simulink model "full_maneuver_single_veh"  (R2020a)
settings: Solver=VariableStepAuto  StartTime=0.0  StopTime=90  FixedStep=0.1  MaxStep=5e-2  RelTol=1e-3
InitFcn:
  | totalVehicles = 5;
  | if exist('vehStatesBus', 'var')==0
  | load vehBuses
  | end
  | if exist('vehErrorsBus', 'var')==0
  | load vehBuses
  | end
libraries: simulink x69, powerlib_meascontrol x6, autolibshared x6, dspsigops x3, eeGeneralControl x2
(part 2 of 6)

== system full_maneuver_single_veh/Lo ==
  allVehicles : Inport
  Constant{,1,3,6} (4 alike) : Constant  Value=0
  Gain : Gain  Gain=m/2
  Regular Vehicle Following : Subsystem
  Terminator{,1..3,9..12} (8 alike) : Terminator
  Transfer Fcn : TransferFcn  Denominator=[tau 1]
  Transport Delay1 : TransportDelay  DelayTime=0.01
  Vehicle Body 3DOF Single Track : autolibshared/Vehicle Body 3DOF Single Track  trackMode=Single (bicycle)  inputMode=External longitudinal forces  frontSteerMode=on  rearSteerMode=off  windMode=off  muMode=off  extFMode=off  extMMode=off  extXo=off  extpsio=off  extxdoto=off  extro=off  extYo=off  extTamb=off  extydoto=off  aMode=2  NF=2  NR=2  m=m  a=lf  b=lr  h=0.35  X_o=x0  xdot_o=vx0  CalphaMode=off  sigmaMode=on  d=0  w=[1.4,1.4]  Cy_f=12e3  Cy_r=11e3  sigma_f=.1  sigma_r=.1  alpha_f_brk=[-.1 .1]  Cy_f_data=[-9e3 9e3]  alpha_r_brk=[-.1 .1]  Cy_r_data=[-9e3 9e3]  Y_o=y0  ydot_o=0  Izz=4000  psi_o=0  r_o=0  Af=2  Cd=.3  Cl=.1  Cpm=.1  beta_w=[0:0.01:0.3]  Cs=[0:0.03:0.9]  Cym=[0:0.01:0.3]  Pabs=101325  Tair=273  g=9.81  mu=1  xdot_tol=.01  Fznom=5000  Fxtire_sat=7e4  Fytire_sat=7e4  longOff=0  latOff=0  vertOff=0  wrapAng=off
      settings: SourceProductBaseCode=PW,MT,VE,VP
  findLeader : Subsystem
  states routing : Subsystem
  states : Outport  VectorParamsAs1DForOutWhenUnconnected=off
  errors : Outport  Port=2  VectorParamsAs1DForOutWhenUnconnected=off
  gap : Outport  Port=3  VectorParamsAs1DForOutWhenUnconnected=off
  wires:
  Transfer Fcn/1 -> Gain/1
  findLeader/1(leader) -> Regular Vehicle Following/2(leader)
  Regular Vehicle Following/4(leaderInRange) -> Terminator3/1
  Constant3/1 -> Regular Vehicle Following/4(extraSpaceFlag)
  Constant/1 -> states routing/1(delta), Vehicle Body 3DOF Single Track/1  "delta"
  Regular Vehicle Following/2(errors) -> errors/1
  Regular Vehicle Following/1(u) -> Transport Delay1/1  "u"
  findLeader/2(leaderChange) -> Regular Vehicle Following/3(leaderChange)
  Transport Delay1/1 -> states routing/3(u), Transfer Fcn/1
  states routing/2(observedStates) -> Regular Vehicle Following/1(ego), findLeader/1(ego), states/1
  Vehicle Body 3DOF Single Track/1 -> states routing/2(Info)
  Gain/1 -> Vehicle Body 3DOF Single Track/3, Vehicle Body 3DOF Single Track/2
  allVehicles/1 -> findLeader/2(all)
  Regular Vehicle Following/3(gap) -> gap/1
  Constant1/1 -> findLeader/4(state)
  Constant6/1 -> findLeader/3(lcFlag)
  states routing/1(latStates) -> Terminator1/1
  Vehicle Body 3DOF Single Track/2 -> Terminator2/1
  Vehicle Body 3DOF Single Track/5 -> Terminator10/1
  Vehicle Body 3DOF Single Track/3 -> Terminator/1
  Vehicle Body 3DOF Single Track/6 -> Terminator11/1
  Vehicle Body 3DOF Single Track/7 -> Terminator12/1
  Vehicle Body 3DOF Single Track/4 -> Terminator9/1

== system full_maneuver_single_veh/Subsystem ==
  note: Lane change not yet completed
  laneChangeIntention : Inport
  platoonState : Inport  Port=2
  AND : Logic  IconShape=distinctive  AllPortsSameDT=off  OutDataTypeStr=boolean
  Compare To Constant : simulink/Logic and Bit Operations/Compare To Constant  relop=<  const=5  OutDataTypeStr=boolean
  Selector : Selector  InputPortWidth=1  IndexOptions=Index vector (dialog)  Indices=[1]  OutputSizes=1
  gapRequest : Outport
  wires:
  laneChangeIntention/1 -> AND/1
  platoonState/1 -> Selector/1
  Selector/1 -> Compare To Constant/1
  AND/1 -> gapRequest/1
  Compare To Constant/1 -> AND/2

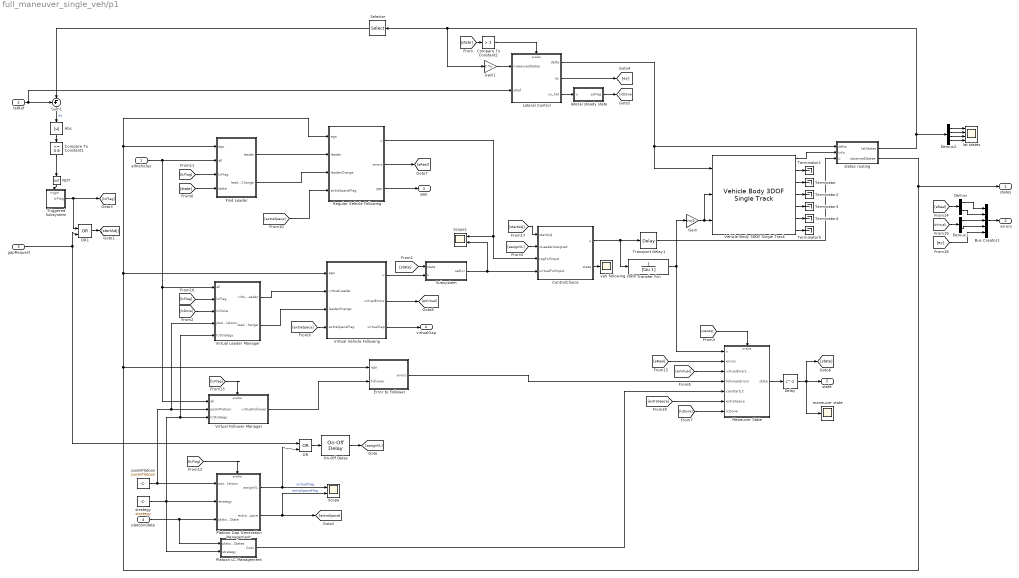
== system full_maneuver_single_veh/p1 ==
  allVehicles : Inport
  latRef : Inport  Port=2
  gapRequest : Inport  Port=3
  platoonState : Inport  Port=4
  Abs : Abs
  Bus Creator1 : BusCreator  Inputs=5  OutDataTypeStr=Bus: vehErrorsBus  NonVirtualBus=on
      settings: InheritFromInputs=off
  Compare To Constant1 : simulink/Logic and Bit Operations/Compare To Constant  relop=<=  const=0.8  OutDataTypeStr=boolean
  Compare To Constant2 : simulink/Logic and Bit Operations/Compare To Constant  relop=>  const=3  OutDataTypeStr=boolean
  ControlChoice : Stateflow chart  TreatAsAtomicUnit=on
  Delay : Delay
  Demux : Demux  Outputs=2
  Demux1 : Demux  Outputs=2
  Demux2 : Demux
  Error to Follower : Subsystem
  Find Leader : Subsystem
  Gain : Gain  Gain=m/2
  Gain1 : Gain  Gain=C  Multiplication=Matrix(K*u)
  Lateral Control : Subsystem
  Maneuver State : Subsystem
  NOT : Logic  Operator=NOT  IconShape=distinctive  AllPortsSameDT=off  OutDataTypeStr=boolean
  OR : Logic  Operator=OR  IconShape=distinctive  AllPortsSameDT=off  OutDataTypeStr=boolean
  OR1 : Logic  Operator=OR  IconShape=distinctive  AllPortsSameDT=off  OutDataTypeStr=boolean
  On-Off Delay : eeGeneralControl/On-Off Delay  LabelModeActiveChoice=Continuous  Td_on=0.1  Td_off=1  IC=0  Ts=0
      settings: SourceProductBaseCode=PS
  Platoon Gap Generation Management : Subsystem
  Platoon LC Management : Subsystem
  Regular Vehicle Following : Subsystem
  Scope : Scope  NumInputPorts=2
  Scope1 : Scope  NumInputPorts=2
  Selector : Selector  InputPortWidth=4  IndexOptions=Index vector (dialog)  Indices=1  OutputSizes=1
  Subsystem : Subsystem
  Sum1 : Sum  Inputs=+-|
  Terminator{,1..5} (6 alike) : Terminator
  Transfer Fcn : TransferFcn  Denominator=[tau 1]
  Transport Delay1 : TransportDelay  DelayTime=0.01
  Triggered Subsystem : Subsystem  TreatAsAtomicUnit=on
  Vehicle Body 3DOF Single Track : autolibshared/Vehicle Body 3DOF Single Track  trackMode=Single (bicycle)  inputMode=External longitudinal forces  frontSteerMode=on  rearSteerMode=off  windMode=off  muMode=off  extFMode=off  extMMode=off  extXo=off  extpsio=off  extxdoto=off  extro=off  extYo=off  extTamb=off  extydoto=off  aMode=2  NF=2  NR=2  m=m  a=lf  b=lr  h=0.35  X_o=x0  xdot_o=vx0  CalphaMode=off  sigmaMode=on  d=0  w=[1.4,1.4]  Cy_f=12e3  Cy_r=11e3  sigma_f=.1  sigma_r=.1  alpha_f_brk=[-.1 .1]  Cy_f_data=[-9e3 9e3]  alpha_r_brk=[-.1 .1]  Cy_r_data=[-9e3 9e3]  Y_o=y0  ydot_o=0  Izz=4000  psi_o=0  r_o=0  Af=2  Cd=.3  Cl=.1  Cpm=.1  beta_w=[0:0.01:0.3]  Cs=[0:0.03:0.9]  Cym=[0:0.01:0.3]  Pabs=101325  Tair=273  g=9.81  mu=1  xdot_tol=.01  Fznom=5000  Fxtire_sat=7e4  Fytire_sat=7e4  longOff=0  latOff=0  vertOff=0  wrapAng=off
      settings: SourceProductBaseCode=PW,MT,VE,VP
  Virtual Follower Manager : Subsystem  TreatAsAtomicUnit=on
  Virtual Leader Manager : Subsystem  TreatAsAtomicUnit=on
  Virtual Vehicle Following : Subsystem  TreatAsAtomicUnit=on
  lat states : Scope  NumInputPorts=4
  lateral steady state : Subsystem
  maneuver state : Scope
  posInPlatoon : Constant  Value=posInPlatoon
  states routing : Subsystem
  strategy : Constant  Value=strategy
  veh following state : Scope
  states : Outport  VectorParamsAs1DForOutWhenUnconnected=off
  errors : Outport  Port=2  VectorParamsAs1DForOutWhenUnconnected=off
  gap : Outport  Port=3  VectorParamsAs1DForOutWhenUnconnected=off
  virtualGap : Outport  Port=4  VectorParamsAs1DForOutWhenUnconnected=off
  state : Outport  Port=5  VectorParamsAs1DForOutWhenUnconnected=off
  wires:
  [extraSpace] -> Maneuver State/6(extraSpace)
  [eReal] -> Maneuver State/2(errors)
  [eVirtual] -> Maneuver State/3(virtualErrors)
  [lcDone] -> Maneuver State/7(lcDone)
  [startAdj] -> Maneuver State/Enable
  Platoon LC Management/1(Out1) -> Maneuver State/5(canStartLC)
  Error to Follower/1(errors) -> Maneuver State/4(followerErrors)
  Maneuver State/1(state) -> Delay/1
  [lcFlag] -> Virtual Leader Manager/2(lcFlag)
  [lcDone] -> Virtual Leader Manager/3(lcDone)
  [lcFlag] -> Virtual Follower Manager/Enable
  [lcFlag] -> Platoon Gap Generation Management/Enable
  [lcFlag] -> Find Leader/3(lcFlag)
  [extraSpace] -> Regular Vehicle Following/4(extraSpaceFlag)
  [extraSpace] -> Virtual Vehicle Following/4(extraSpaceFlag)
  Platoon Gap Generation Management/1(assignVL) -> OR/2, Scope/1  "virtualFlag"
  [assignVL] -> ControlChoice/2(vLeaderAssigned)
  gapRequest/1 -> OR/1, OR1/2
  Triggered Subsystem/1(lcFlag) -> [lcFlag], OR1/1
  Regular Vehicle Following/2(errors) -> [eReal]
  Virtual Vehicle Following/2(virtualErrors) -> [eVirtual]
  Virtual Leader Manager/2(leaderChange) -> Virtual Vehicle Following/3(leaderChange)
  Compare To Constant1/1 -> NOT/1
  [startAdj] -> ControlChoice/1(startAdj)
  Virtual Leader Manager/1(virtualLeader) -> Virtual Vehicle Following/2(virtualLeader)
  posInPlatoon/1 -> Virtual Leader Manager/4(posInPlatoon), Virtual Follower Manager/2(posInPlatoon), Platoon Gap Generation Management/1(posInPlatoon)
  [state] -> Subsystem/1(state)
  Find Leader/1(leader) -> Regular Vehicle Following/2(leader)
  Subsystem/1(sat(u)) -> ControlChoice/4(virtualFollInput), Scope1/2
  Find Leader/2(leaderChange) -> Regular Vehicle Following/3(leaderChange)
  Sum1/1 -> Abs/1  "ey"
  Transfer Fcn/1 -> Gain/1, Maneuver State/1(u)
  states routing/2(observedStates) -> states/1, Virtual Vehicle Following/1(ego), Regular Vehicle Following/1(ego), Find Leader/1(ego), Error to Follower/1(ego)
  latRef/1 -> Lateral Control/2(yRef), Sum1/1
  Vehicle Body 3DOF Single Track/3 -> Terminator/1
  Vehicle Body 3DOF Single Track/1 -> states routing/2(Info)
  Gain/1 -> Vehicle Body 3DOF Single Track/3, Vehicle Body 3DOF Single Track/2
  Platoon Gap Generation Management/2(extraSpace) -> Scope/2, [extraSpace]  "extraSpaceFlag"
  Abs/1 -> Compare To Constant1/1
  allVehicles/1 -> Find Leader/2(all), Virtual Leader Manager/1(all), Virtual Follower Manager/1(all)
  Regular Vehicle Following/3(gap) -> gap/1
  Regular Vehicle Following/1(u) -> ControlChoice/3(regFollInput), Scope1/1
  Virtual Vehicle Following/1(u) -> Subsystem/2(u)
  Compare To Constant2/1 -> Lateral Control/Enable
  Virtual Vehicle Following/3(virtualGap) -> virtualGap/1
  [state] -> Compare To Constant2/1
  platoonState/1 -> Platoon Gap Generation Management/3(platoonState), Platoon LC Management/1(platoonStates)
  Delay/1 -> state/1, [state], maneuver state/1
  strategy/1 -> Virtual Leader Manager/5(lcStrategy), Virtual Follower Manager/3(lcStrategy), Platoon LC Management/2(strategy), Platoon Gap Generation Management/2(strategy)
  [state] -> Find Leader/4(state)
  OR1/1 -> [startAdj]
  states routing/1(latStates) -> Demux2/1, Selector/1, Gain1/1
  Gain1/1 -> Lateral Control/1(measuredStates)
  NOT/1 -> Triggered Subsystem/Trigger
  Lateral Control/3(vy_hat) -> lateral steady state/1(u)
  lateral steady state/1(ssFlag) -> [lcDone]
  Lateral Control/2(ey) -> [ey]
  [eVirtual] -> Demux1/1
  [eReal] -> Demux/1
  Demux/1 -> Bus Creator1/1
  Demux/2 -> Bus Creator1/2
  Demux1/1 -> Bus Creator1/3
  Demux1/2 -> Bus Creator1/4
  [ey] -> Bus Creator1/5
  Bus Creator1/1 -> errors/1
  OR/1 -> On-Off Delay/1
  Lateral Control/1(delta) -> Vehicle Body 3DOF Single Track/1, states routing/1(delta)
  Demux2/1 -> lat states/1
  Demux2/2 -> lat states/2
  Demux2/3 -> lat states/3
  Demux2/4 -> lat states/4
  Selector/1 -> Sum1/2
  Vehicle Body 3DOF Single Track/2 -> Terminator1/1
  Vehicle Body 3DOF Single Track/4 -> Terminator2/1
  Vehicle Body 3DOF Single Track/5 -> Terminator3/1
  Vehicle Body 3DOF Single Track/6 -> Terminator4/1
  Vehicle Body 3DOF Single Track/7 -> Terminator5/1
  ControlChoice/1(u) -> Transfer Fcn/1, Transport Delay1/1
  Virtual Follower Manager/1(virtualFollower) -> Error to Follower/2(follower)
  ControlChoice/2(state) -> veh following state/1
  Transport Delay1/1 -> states routing/3(u)
  On-Off Delay/1 -> [assignVL]

== system full_maneuver_single_veh/Fd/Error to Follower ==
  ego : Inport
  follower : Inport  Port=2
  Bus Selector : BusSelector  OutputSignals=X,Xdot
  Bus Selector1 : BusSelector  OutputSignals=X,Xdot
  Multiply : Product
  Mux : Mux  Inputs=2
  Sum : Sum  Inputs=-+|
  Sum1 : Sum  Inputs=++|
  Sum2 : Sum  Inputs=+-|
  Sum3 : Sum  Inputs=|++
  Sum4 : Sum  Inputs=-+|
  d0 : Constant  Value=d0
  h : Constant  Value=h
  vLen : Constant  Value=lr+lf
  errors : Outport  VectorParamsAs1DForOutWhenUnconnected=off
  wires:
  d0/1 -> Sum3/2  "gap at  standstill"
  h/1 -> Multiply/2  "time headway"
  Sum2/1 -> Mux/1
  Bus Selector1/1 -> Sum/2  "<X>"
  Sum1/1 -> Sum/1  "x (front bumber)"
  Sum3/1 -> Sum2/2  "desired  gap"
  Bus Selector/1 -> Sum1/2  "<X>"
  Sum/1 -> Sum2/1  "gap"
  Multiply/1 -> Sum3/1
  vLen/1 -> Sum1/1
  follower/1 -> Bus Selector/1
  ego/1 -> Bus Selector1/1
  Bus Selector/2 -> Sum4/1, Multiply/1  "<Xdot>"
  Bus Selector1/2 -> Sum4/2  "<Xdot>"
  Sum4/1 -> Mux/2
  Mux/1 -> errors/1

== system full_maneuver_single_veh/Fd/Find Leader ==
  ego : Inport
  all : Inport  Port=2
  lcFlag : Inport  Port=3
  state : Inport  Port=4
  Compare To Constant : simulink/Logic and Bit Operations/Compare To Constant  relop=~=  const=4  OutDataTypeStr=boolean
  Detect Change : simulink/Logic and Bit Operations/Detect Change  vinit=0  OutDataTypeStr=boolean
  NOT : Logic  Operator=NOT  IconShape=distinctive  AllPortsSameDT=off  OutDataTypeStr=boolean
  OR : Logic  Operator=OR  IconShape=distinctive  AllPortsSameDT=off  OutDataTypeStr=boolean
  Selector : Selector  InputPortWidth=totalVehicles+1  IndexOptions=Index vector (port)  Indices=[1]  OutputSizes=1
  Subsystem : Subsystem
  Vector Concatenate : Concatenate
  farAwayVeh : Subsystem
  realLeaderIdx : Scope
  leader : Outport  VectorParamsAs1DForOutWhenUnconnected=off
  leaderChange : Outport  Port=2  InitialOutput=1  VectorParamsAs1DForOutWhenUnconnected=off
  wires:
  Compare To Constant/1 -> OR/2
  state/1 -> Compare To Constant/1
  ego/1 -> Subsystem/1(ego), farAwayVeh/1(ego)
  all/1 -> Vector Concatenate/1, Subsystem/2(all)
  Subsystem/1(idx) -> realLeaderIdx/1, Selector/2, Detect Change/1
  OR/1 -> Subsystem/Enable
  lcFlag/1 -> NOT/1
  NOT/1 -> OR/1
  Selector/1 -> leader/1
  farAwayVeh/1(Out1) -> Vector Concatenate/2
  Vector Concatenate/1 -> Selector/1
  Detect Change/1 -> leaderChange/1

== system full_maneuver_single_veh/Fd/Lateral Control ==
  measuredStates : Inport
  yRef : Inport  Port=2
  Enable : EnablePort
  Demux2 : Demux
  Full State Observer : Subsystem  Commented=on
  Gain : Gain  Gain=5
  Gain1 : Gain  Gain=Klat  Multiplication=Matrix(K*u)
  Integrator : Integrator  InitialCondition=y0
  Pad : dspsigops/Pad  padAlong=Columns  dimsToPad=1  valSrc=Specify via dialog  padVal=0  spec=Output size  padNumOutRowsSpecMethod=User-specified  numOutRows=4  padNumOutColsSpecMethod=User-specified  numOutCols=1  isVarDimsMode=off  padBeginning=0  padEnd=0  outSizeMode=User-specified  outSize=1  padSigAt=End  trunc_flag=None  roundingMode=Floor  overflowMode=off  truncOrWrapMode=Truncate  wrap_flag=None
      settings: SourceProductBaseCode=DS
  Rate Limiter : RateLimiter  RisingSlewLimit=maxDeltaDot  FallingSlewLimit=-maxDeltaDot  SampleTimeMode=inherited
  Saturation : Saturate  UpperLimit=maxDelta  LowerLimit=-maxDelta
  Saturation1 : Saturate  UpperLimit=2  LowerLimit=-2
  Scope : Scope  NumInputPorts=4
  Scope1 : Scope  NumInputPorts=2
  Selector : Selector  InputPortWidth=4  IndexOptions=Index vector (dialog)  Indices=[1]  OutputSizes=1
  Sum : Sum  Inputs=|+-
  Sum2 : Sum  Inputs=|+-
  delta : Outport  VectorParamsAs1DForOutWhenUnconnected=off
  ey : Outport  Port=2  VectorParamsAs1DForOutWhenUnconnected=off
  vy_hat : Outport  Port=3  InitialOutput=0.3  VectorParamsAs1DForOutWhenUnconnected=off
  wires:
  Selector/1 -> ey/1
  Saturation1/1 -> Integrator/1
  Gain/1 -> Saturation1/1
  measuredStates/1 -> Sum/2, Demux2/1, Full State Observer/1(measuredOutputs)  "estStates"
  yRef/1 -> Sum2/1
  Demux2/3 -> Scope/3
  Saturation/1 -> Rate Limiter/1
  Sum2/1 -> Gain/1
  Demux2/2 -> Scope/2, vy_hat/1
  Demux2/4 -> Scope/4
  Pad/1 -> Sum/1
  Sum/1 -> Gain1/1, Selector/1
  Gain1/1 -> Saturation/1, Scope1/2
  Integrator/1 -> Pad/1, Sum2/2
  Demux2/1 -> Scope/1
  Rate Limiter/1 -> delta/1, Scope1/1, Full State Observer/2(delta)  "delta"

== system full_maneuver_single_veh/Fd/Maneuver State ==
  note: States are:
      | 0 - Lane keeping
      | 1 - Longitudinal Adjustment
      | 2 - Steady State
      | 3 - Safe to LC
      | 4 - Performing LC
      | 5 - LC is done
      | 6 - Long Adj done
  u : Inport
  errors : Inport  Port=2
  virtualErrors : Inport  Port=3
  followerErrors : Inport  Port=4
  canStartLC : Inport  Port=5
  extraSpace : Inport  Port=6
  lcDone : Inport  Port=7
  Enable : EnablePort
  AND : Logic  IconShape=distinctive  AllPortsSameDT=off  OutDataTypeStr=boolean
  AND1 : Logic  IconShape=distinctive  AllPortsSameDT=off  OutDataTypeStr=boolean
  AND2 : Logic  Inputs=3  IconShape=distinctive  AllPortsSameDT=off  OutDataTypeStr=boolean
  AND{3..7} (5 alike) : Logic  IconShape=distinctive  AllPortsSameDT=off  OutDataTypeStr=fixdt(1,16)
  Constant : Constant
  Data Type Conversion : DataTypeConversion  OutMin=0  OutMax=1  OutDataTypeStr=fixdt(1,16)
  Memory : Memory
  NOT1 : Logic  Operator=NOT  IconShape=distinctive  AllPortsSameDT=off  OutDataTypeStr=boolean
  On Delay : powerlib_meascontrol/Logic/On Delay  DelayType=On delay  delay=1  ic=0  Ts=0
  On Delay1 : powerlib_meascontrol/Logic/On Delay  DelayType=On delay  delay=0.2  ic=0  Ts=0
  Scope : Scope  NumInputPorts=5
  Sum : Sum  Inputs=++++++
  Triggered Subsystem : Subsystem  TreatAsAtomicUnit=on
  Triggered Subsystem1 : Subsystem  TreatAsAtomicUnit=on
  safeErrors : Subsystem
  safeErrors1 : Subsystem
  safeErrors2 : Subsystem
  steadyState : Subsystem
  state : Outport  InitialOutput=0  VectorParamsAs1DForOutWhenUnconnected=off
  wires:
  u/1 -> steadyState/1(u)
  AND1/1 -> AND/1, AND2/1  "steady state"
  steadyState/1(ssFlag) -> AND1/1
  safeErrors2/1(safetyFlag) -> AND2/2
  Triggered Subsystem1/1(Out1) -> Memory/1
  NOT1/1 -> On Delay1/1
  On Delay/1 -> AND2/3
  extraSpace/1 -> On Delay/1, NOT1/1
  safeErrors1/1(safetyFlag) -> AND1/2
  AND2/1 -> Triggered Subsystem1/Trigger
  On Delay1/1 -> AND/2
  followerErrors/1 -> safeErrors/1(errors)
  errors/1 -> safeErrors1/1(errors)
  virtualErrors/1 -> safeErrors2/1(errors)
  Triggered Subsystem/1(Out1) -> Sum/6
  canStartLC/1 -> AND5/2
  lcDone/1 -> AND6/2
  AND7/1 -> Scope/5, Triggered Subsystem/Trigger
  Data Type Conversion/1 -> Sum/1
  AND/1 -> AND7/2
  AND6/1 -> AND7/1, Sum/5, Scope/4
  Constant/1 -> AND3/1, Data Type Conversion/1
  AND5/1 -> Sum/4, Scope/3, AND6/1
  AND3/1 -> Sum/2, Scope/1, AND4/1
  Sum/1 -> state/1
  safeErrors/1(safetyFlag) -> AND4/2
  AND4/1 -> Sum/3, Scope/2, AND5/1
  Memory/1 -> AND3/2

== system full_maneuver_single_veh/Fd/Platoon Gap Generation Management ==
  posInPlatoon : Inport
  strategy : Inport  Port=2
  platoonState : Inport  Port=3
  Enable : EnablePort
  Scope : Scope  NumInputPorts=2
  assignExtraSpace : MATLAB Function  TreatAsAtomicUnit=on
  assignvirtualLeader : MATLAB Function  TreatAsAtomicUnit=on
  assignVL : Outport  VectorParamsAs1DForOutWhenUnconnected=off
  extraSpace : Outport  Port=2  VectorParamsAs1DForOutWhenUnconnected=off
  wires:
  assignvirtualLeader/1(virtualLeaderFlag) -> assignVL/1, Scope/1
  platoonState/1 -> assignExtraSpace/3(platoonState), assignvirtualLeader/3(platoonState)
  posInPlatoon/1 -> assignExtraSpace/2(posInPlatoon), assignvirtualLeader/2(posInPlatoon)
  strategy/1 -> assignExtraSpace/1(strategy), assignvirtualLeader/1(strategy)
  assignExtraSpace/1(extraSpaceFlag) -> extraSpace/1, Scope/2

== system full_maneuver_single_veh/Fd/Platoon LC Management ==
  platoonStates : Inport
  strategy : Inport  Port=2
  Compare To Constant : simulink/Logic and Bit Operations/Compare To Constant  relop=>  const=1  OutDataTypeStr=boolean
  Compare To Constant1 : simulink/Logic and Bit Operations/Compare To Constant  relop=>  const=2  OutDataTypeStr=boolean
  OR : Logic  Operator=OR  IconShape=distinctive  AllPortsSameDT=off  OutDataTypeStr=boolean
  Selector : Selector  IndexOptions=Index vector (port)  Indices=[1 3]  OutputSizes=1
  Width : Width
  Out1 : Outport  VectorParamsAs1DForOutWhenUnconnected=off
  wires:
  Compare To Constant1/1 -> OR/1
  Selector/1 -> Compare To Constant1/1
  Width/1 -> Selector/2
  platoonStates/1 -> Selector/1, Width/1
  OR/1 -> Out1/1
  Compare To Constant/1 -> OR/2
  strategy/1 -> Compare To Constant/1

== system full_maneuver_single_veh/Fd/Regular Vehicle Following ==
  ego : Inport
  leader : Inport  Port=2
  leaderChange : Inport  Port=3
  extraSpaceFlag : Inport  Port=4
  Bus Selector : BusSelector  OutputSignals=u
  Compute Errors : Subsystem
  Constant : Constant  Value=0
  Define Desired Distance : Subsystem
  Rate Limiter : RateLimiter  RisingSlewLimit=maxJerk  FallingSlewLimit=minJerk  SampleTimeMode=inherited
  Rate Limiter1 : RateLimiter  RisingSlewLimit=maxComfJerk  FallingSlewLimit=minComfJerk  SampleTimeMode=inherited
  Switch : Switch  Criteria=u2 > Threshold
  Switch1 : Switch  Criteria=u2 > Threshold
  Veh Following : Subsystem  TreatAsAtomicUnit=on
  Velocity Control : Subsystem  TreatAsAtomicUnit=on
  Velocity Error : Subsystem
  comf saturation : Saturate  UpperLimit=maxComfAccel  LowerLimit=minComfAccel
  errorScope : Scope
  freeFlowVel : Constant  Value=freeFlowVel
  safe saturation : Saturate  UpperLimit=maxAcceleration  LowerLimit=minAcceleration
  switch free flow : Subsystem
  veh foll state : Scope  NumInputPorts=2
  u : Outport  VectorParamsAs1DForOutWhenUnconnected=off
  errors : Outport  Port=2  VectorParamsAs1DForOutWhenUnconnected=off
  gap : Outport  Port=3  VectorParamsAs1DForOutWhenUnconnected=off
  wires:
  extraSpaceFlag/1 -> Define Desired Distance/1(extraSpaceFlag), Velocity Error/3(filterReset)
  switch free flow/1(inRange) -> Switch/2, veh foll state/1, Veh Following/5(inRange)
  Velocity Error/1(ev) -> Velocity Control/1(ev)
  Velocity Error/2(ea) -> Velocity Control/2(ea)
  leaderChange/1 -> Veh Following/4(leaderChange)
  Veh Following/1(u) -> Switch/1
  Constant/1 -> Compute Errors/5(velFilterReset)
  leader/1 -> Compute Errors/2(leader)
  Compute Errors/1(errors) -> switch free flow/1(errors), Veh Following/1(errors), errors/1, errorScope/1
  comf saturation/1 -> Rate Limiter1/1
  safe saturation/1 -> Rate Limiter/1
  Rate Limiter/1 -> Switch1/1  "sat(u)"
  Switch1/1 -> u/1
  Switch/1 -> veh foll state/2, safe saturation/1, comf saturation/1
  Rate Limiter1/1 -> Switch1/3  "sat(u)"
  Compute Errors/3("gap ") -> gap/1, switch free flow/3(gap)
  ego/1 -> Compute Errors/1(ego), Bus Selector/1, Velocity Error/1(ego)
  Velocity Control/1(u) -> Switch/3
  freeFlowVel/1 -> Velocity Error/2(velRef), switch free flow/6(vRef)
  Compute Errors/4(unsafeFlag) -> Switch1/2
  Bus Selector/1 -> Veh Following/3(realInput), Velocity Control/3(realInput)  "<u>"
  Compute Errors/2(errorsDot) -> Veh Following/2(errorsDot), switch free flow/2(errorsDot)
  Define Desired Distance/1(h) -> Compute Errors/3(h), switch free flow/4(h)
  Define Desired Distance/2(d0) -> Compute Errors/4(d0), switch free flow/5(d0)

== system full_maneuver_single_veh/Fd/Subsystem ==
  state : Inport
  u : Inport  Port=2
  Compare To Constant : simulink/Logic and Bit Operations/Compare To Constant  relop===  const=7  OutDataTypeStr=boolean
  Scope : Scope
  Switch1 : Switch  Criteria=u2 > Threshold
  comf saturation : Saturate  UpperLimit=maxComfAccel  LowerLimit=minComfAccel
  comf jerk : RateLimiter  RisingSlewLimit=maxComfJerk  FallingSlewLimit=minComfJerk  SampleTimeMode=inherited
  safe saturation : Saturate  UpperLimit=maxAcceleration  LowerLimit=minAcceleration
  safe jerk : RateLimiter  RisingSlewLimit=maxJerk  FallingSlewLimit=minJerk  SampleTimeMode=inherited
  sat(u) : Outport  VectorParamsAs1DForOutWhenUnconnected=off
  wires:
  safe saturation/1 -> safe jerk/1
  safe jerk/1 -> Switch1/1
  comf saturation/1 -> comf jerk/1
  state/1 -> Compare To Constant/1
  u/1 -> comf saturation/1, safe saturation/1
  comf jerk/1 -> Switch1/3
  Switch1/1 -> Scope/1, sat(u)/1
  Compare To Constant/1 -> Switch1/2

== system full_maneuver_single_veh/Fd/Triggered Subsystem ==
  Trigger : TriggerPort  VariantControl=Variant
  Constant : Constant
  lcFlag : Outport  InitialOutput=0  VectorParamsAs1DForOutWhenUnconnected=off
  wires:
  Constant/1 -> lcFlag/1

== system full_maneuver_single_veh/Fd/Virtual Follower Manager ==
  all : Inport
  posInPlatoon : Inport  Port=2
  lcStrategy : Inport  Port=3
  Enable : EnablePort
  Selector1 : Selector  InputPortWidth=totalVehicles  IndexOptions=Index vector (port)  Indices=[1]  OutputSizes=1
  Width : Width
  determineVirtualFollower : MATLAB Function  TreatAsAtomicUnit=on
  virtualFollower : Outport
  wires:
  Width/1 -> determineVirtualFollower/1(nVehicles)
  lcStrategy/1 -> determineVirtualFollower/3(lcStrategy)
  determineVirtualFollower/1(virtualFollowerIdx) -> Selector1/2
  posInPlatoon/1 -> determineVirtualFollower/2(posInPlatoon)
  all/1 -> Selector1/1, Width/1
  Selector1/1 -> virtualFollower/1

== system full_maneuver_single_veh/Fd/Virtual Leader Manager ==
  all : Inport
  lcFlag : Inport  Port=2
  lcDone : Inport  Port=3
  posInPlatoon : Inport  Port=4
  lcStrategy : Inport  Port=5
  Detect Change : simulink/Logic and Bit Operations/Detect Change  vinit=0  OutDataTypeStr=boolean
  Selector : Selector  InputPortWidth=totalVehicles  IndexOptions=Index vector (port)  Indices=[1]  OutputSizes=1
  Width : Width
  determineVirtualLeader : MATLAB Function  TreatAsAtomicUnit=on
  virtualVehs : Scope
  virtualLeader : Outport  VectorParamsAs1DForOutWhenUnconnected=off
  leaderChange : Outport  Port=2  VectorParamsAs1DForOutWhenUnconnected=off
  wires:
  all/1 -> Selector/1, Width/1
  Selector/1 -> virtualLeader/1
  Detect Change/1 -> leaderChange/1
  determineVirtualLeader/1(virtualLeaderIdx) -> Selector/2, Detect Change/1, virtualVehs/1
  Width/1 -> determineVirtualLeader/1(nVehicles)
  lcFlag/1 -> determineVirtualLeader/2(lcFlag)
  lcDone/1 -> determineVirtualLeader/3(lcDone)
  posInPlatoon/1 -> determineVirtualLeader/4(posInPlatoon)
  lcStrategy/1 -> determineVirtualLeader/5(lcStrategy)

== system full_maneuver_single_veh/Fd/Virtual Vehicle Following ==
  ego : Inport
  virtualLeader : Inport  Port=2
  leaderChange : Inport  Port=3
  extraSpaceFlag : Inport  Port=4
  Bus Selector : BusSelector  OutputSignals=u
  Compute Errors : Subsystem
  Define Desired Distance : Subsystem
  Min Velocity Control : Subsystem  TreatAsAtomicUnit=on
  Min Velocity Error : Subsystem
  NOT : Logic  Operator=NOT  IconShape=distinctive  AllPortsSameDT=off  OutDataTypeStr=boolean
  Scope : Scope  NumInputPorts=2
  Switch : Switch  Criteria=u2 > Threshold
  Terminator : Terminator
  Virtual Leader Following : Subsystem  TreatAsAtomicUnit=on
  switch min vel : Subsystem
  vMin : Constant  Value=vMin
  u : Outport  InitialOutput=0  VectorParamsAs1DForOutWhenUnconnected=off
  virtualErrors : Outport  Port=2  OutputWhenDisabled=reset  InitialOutput=[0, 0]  VectorParamsAs1DForOutWhenUnconnected=off
  virtualGap : Outport  Port=3  OutputWhenDisabled=reset  InitialOutput=[0]  VectorParamsAs1DForOutWhenUnconnected=off
  wires:
  Bus Selector/1 -> Min Velocity Control/3(realInput), Virtual Leader Following/3(realInput)  "<u>"
  Min Velocity Error/2(ea) -> Min Velocity Control/2(ea)
  Min Velocity Error/1(ev) -> Min Velocity Control/1(ev)
  NOT/1 -> Switch/2, Scope/1, Virtual Leader Following/5(inRange)
  switch min vel/1(inRange) -> NOT/1, Min Velocity Error/3(filterReset)
  extraSpaceFlag/1 -> Define Desired Distance/1(extraSpaceFlag)
  Min Velocity Control/1(u) -> Switch/3  "uMinVelControl"
  Compute Errors/3("gap ") -> virtualGap/1, switch min vel/3(gap)
  Virtual Leader Following/1(u) -> Switch/1  "uVehFoll"
  ego/1 -> Compute Errors/1(ego), Min Velocity Error/1(ego), Bus Selector/1
  vMin/1 -> Min Velocity Error/2(velRef), switch min vel/6(vRef)
  Compute Errors/1(errors) -> switch min vel/1(errors), Virtual Leader Following/1(errors), virtualErrors/1
  virtualLeader/1 -> Compute Errors/2(leader)
  Switch/1 -> Scope/2, u/1
  leaderChange/1 -> Compute Errors/5(velFilterReset), Virtual Leader Following/4(leaderChange)
  Compute Errors/4(unsafeFlag) -> Terminator/1
  Compute Errors/2(errorsDot) -> Virtual Leader Following/2(errorsDot), switch min vel/2(errorsDot)
  Define Desired Distance/1(h) -> switch min vel/4(h), Compute Errors/3(h)
  Define Desired Distance/2(d0) -> switch min vel/5(d0), Compute Errors/4(d0)

== system full_maneuver_single_veh/Fd/lateral steady state ==
  u : Inport
  AND : Logic  IconShape=distinctive  AllPortsSameDT=off  OutDataTypeStr=boolean
  Abs2 : Abs
  Compare To Constant2 : simulink/Logic and Bit Operations/Compare To Constant  relop=<=  const=0.2  OutDataTypeStr=boolean
  Demux : Demux  Outputs=2
  Mux : Mux  Inputs=2
  Transport Delay2 : TransportDelay
  ssFlag : Outport  VectorParamsAs1DForOutWhenUnconnected=off
  wires:
  u/1 -> Transport Delay2/1, Mux/2
  Abs2/1 -> Compare To Constant2/1
  Demux/1 -> AND/1
  Transport Delay2/1 -> Mux/1
  AND/1 -> ssFlag/1
  Compare To Constant2/1 -> Demux/1
  Mux/1 -> Abs2/1
  Demux/2 -> AND/2

== system full_maneuver_single_veh/Fd/states routing ==
  delta : Inport
  Info : Inport  Port=2
  u : Inport  Port=3
  Bus Creator : BusCreator  Inputs=7  OutDataTypeStr=Bus: vehStatesBus  NonVirtualBus=on
      settings: InheritFromInputs=off
  Bus Selector : BusSelector  OutputSignals=BdyFrm.Cg.Vel.ydot,BdyFrm.Cg.AngVel.r,InertFrm.RearAxl.Disp.X,InertFrm.Cg.Disp.Y,InertFrm.RearAxl.Vel.Xdot,BdyFrm.Cg.Acc.xddot,InertFrm.Cg.Ang.psi
  Mux : Mux
  latStates : Outport
  observedStates : Outport  Port=2
  wires:
  Bus Creator/1 -> observedStates/1
  Bus Selector/2 -> Mux/4  "<r>"
  Bus Selector/1 -> Mux/2  "<ydot>"
  Mux/1 -> latStates/1
  delta/1 -> Bus Creator/7
  u/1 -> Bus Creator/6
  Bus Selector/7 -> Mux/3, Bus Creator/5  "<psi>"
  Bus Selector/6 -> Bus Creator/4  "<xddot>"
  Bus Selector/5 -> Bus Creator/3  "<Xdot>"
  Bus Selector/4 -> Mux/1, Bus Creator/2  "<Y>"
  Bus Selector/3 -> Bus Creator/1  "<X>"
  Info/1 -> Bus Selector/1

== system full_maneuver_single_veh/Fd_bkp/Error to Follower ==
  ego : Inport
  follower : Inport  Port=2
  Bus Selector : BusSelector  OutputSignals=X,Xdot
  Bus Selector1 : BusSelector  OutputSignals=X,Xdot
  Multiply : Product
  Mux : Mux  Inputs=2
  Sum : Sum  Inputs=-+|
  Sum1 : Sum  Inputs=++|
  Sum2 : Sum  Inputs=+-|
  Sum3 : Sum  Inputs=|++
  Sum4 : Sum  Inputs=-+|
  d0 : Constant  Value=d0
  h : Constant  Value=h
  vLen : Constant  Value=lr+lf
  errors : Outport  VectorParamsAs1DForOutWhenUnconnected=off
  wires:
  d0/1 -> Sum3/2  "gap at  standstill"
  h/1 -> Multiply/2  "time headway"
  Sum2/1 -> Mux/1
  Bus Selector1/1 -> Sum/2  "<X>"
  Sum1/1 -> Sum/1  "x (front bumber)"
  Sum3/1 -> Sum2/2  "desired  gap"
  Bus Selector/1 -> Sum1/2  "<X>"
  Sum/1 -> Sum2/1  "gap"
  Multiply/1 -> Sum3/1
  vLen/1 -> Sum1/1
  follower/1 -> Bus Selector/1
  ego/1 -> Bus Selector1/1
  Bus Selector/2 -> Sum4/1, Multiply/1  "<Xdot>"
  Bus Selector1/2 -> Sum4/2  "<Xdot>"
  Sum4/1 -> Mux/2
  Mux/1 -> errors/1

== system full_maneuver_single_veh/Fd_bkp/Find Leader ==
  ego : Inport
  all : Inport  Port=2
  lcFlag : Inport  Port=3
  state : Inport  Port=4
  Compare To Constant : simulink/Logic and Bit Operations/Compare To Constant  relop=~=  const=4  OutDataTypeStr=boolean
  Detect Change : simulink/Logic and Bit Operations/Detect Change  vinit=0  OutDataTypeStr=boolean
  NOT : Logic  Operator=NOT  IconShape=distinctive  AllPortsSameDT=off  OutDataTypeStr=boolean
  OR : Logic  Operator=OR  IconShape=distinctive  AllPortsSameDT=off  OutDataTypeStr=boolean
  Selector : Selector  InputPortWidth=totalVehicles+1  IndexOptions=Index vector (port)  Indices=[1]  OutputSizes=1
  Subsystem : Subsystem
  Vector Concatenate : Concatenate
  farAwayVeh : Subsystem
  realLeaderIdx : Scope
  leader : Outport  VectorParamsAs1DForOutWhenUnconnected=off
  leaderChange : Outport  Port=2  InitialOutput=1  VectorParamsAs1DForOutWhenUnconnected=off
  wires:
  Compare To Constant/1 -> OR/2
  state/1 -> Compare To Constant/1
  ego/1 -> Subsystem/1(ego), farAwayVeh/1(ego)
  all/1 -> Vector Concatenate/1, Subsystem/2(all)
  Subsystem/1(idx) -> realLeaderIdx/1, Selector/2, Detect Change/1
  OR/1 -> Subsystem/Enable
  lcFlag/1 -> NOT/1
  NOT/1 -> OR/1
  Selector/1 -> leader/1
  farAwayVeh/1(Out1) -> Vector Concatenate/2
  Vector Concatenate/1 -> Selector/1
  Detect Change/1 -> leaderChange/1

== system full_maneuver_single_veh/Fd_bkp/Lateral Control ==
  measuredStates : Inport
  yRef : Inport  Port=2
  Enable : EnablePort
  Demux2 : Demux
  Full State Observer : Subsystem  Commented=on
  Gain : Gain  Gain=5
  Gain1 : Gain  Gain=Klat  Multiplication=Matrix(K*u)
  Integrator : Integrator  InitialCondition=y0
  Pad : dspsigops/Pad  padAlong=Columns  dimsToPad=1  valSrc=Specify via dialog  padVal=0  spec=Output size  padNumOutRowsSpecMethod=User-specified  numOutRows=4  padNumOutColsSpecMethod=User-specified  numOutCols=1  isVarDimsMode=off  padBeginning=0  padEnd=0  outSizeMode=User-specified  outSize=1  padSigAt=End  trunc_flag=None  roundingMode=Floor  overflowMode=off  truncOrWrapMode=Truncate  wrap_flag=None
      settings: SourceProductBaseCode=DS
  Rate Limiter : RateLimiter  RisingSlewLimit=maxDeltaDot  FallingSlewLimit=-maxDeltaDot  SampleTimeMode=inherited
  Saturation : Saturate  UpperLimit=maxDelta  LowerLimit=-maxDelta
  Saturation1 : Saturate  UpperLimit=2  LowerLimit=-2
  Scope : Scope  NumInputPorts=4
  Scope1 : Scope  NumInputPorts=2
  Selector : Selector  InputPortWidth=4  IndexOptions=Index vector (dialog)  Indices=[1]  OutputSizes=1
  Sum : Sum  Inputs=|+-
  Sum2 : Sum  Inputs=|+-
  delta : Outport  VectorParamsAs1DForOutWhenUnconnected=off
  ey : Outport  Port=2  VectorParamsAs1DForOutWhenUnconnected=off
  vy_hat : Outport  Port=3  InitialOutput=0.3  VectorParamsAs1DForOutWhenUnconnected=off
  wires:
  Selector/1 -> ey/1
  Saturation1/1 -> Integrator/1
  Gain/1 -> Saturation1/1
  measuredStates/1 -> Sum/2, Demux2/1, Full State Observer/1(measuredOutputs)  "estStates"
  yRef/1 -> Sum2/1
  Demux2/3 -> Scope/3
  Saturation/1 -> Rate Limiter/1
  Sum2/1 -> Gain/1
  Demux2/2 -> Scope/2, vy_hat/1
  Demux2/4 -> Scope/4
  Pad/1 -> Sum/1
  Sum/1 -> Gain1/1, Selector/1
  Gain1/1 -> Saturation/1, Scope1/2
  Integrator/1 -> Pad/1, Sum2/2
  Demux2/1 -> Scope/1
  Rate Limiter/1 -> delta/1, Scope1/1, Full State Observer/2(delta)  "delta"

== system full_maneuver_single_veh/Fd_bkp/Maneuver State ==
  note: States are:
      | 0 - Lane keeping
      | 1 - Longitudinal Adjustment
      | 2 - Steady State
      | 3 - Safe to LC
      | 4 - Performing LC
      | 5 - LC is done
      | 6 - Long Adj done
  u : Inport
  errors : Inport  Port=2
  virtualErrors : Inport  Port=3
  followerErrors : Inport  Port=4
  canStartLC : Inport  Port=5
  extraSpace : Inport  Port=6
  lcDone : Inport  Port=7
  Enable : EnablePort
  AND : Logic  IconShape=distinctive  AllPortsSameDT=off  OutDataTypeStr=boolean
  AND1 : Logic  IconShape=distinctive  AllPortsSameDT=off  OutDataTypeStr=boolean
  AND2 : Logic  Inputs=3  IconShape=distinctive  AllPortsSameDT=off  OutDataTypeStr=boolean
  AND{3..7} (5 alike) : Logic  IconShape=distinctive  AllPortsSameDT=off  OutDataTypeStr=fixdt(1,16)
  Constant : Constant
  Data Type Conversion : DataTypeConversion  OutMin=0  OutMax=1  OutDataTypeStr=fixdt(1,16)
  Memory : Memory
  NOT1 : Logic  Operator=NOT  IconShape=distinctive  AllPortsSameDT=off  OutDataTypeStr=boolean
  On Delay : powerlib_meascontrol/Logic/On Delay  DelayType=On delay  delay=1  ic=0  Ts=0
  On Delay1 : powerlib_meascontrol/Logic/On Delay  DelayType=On delay  delay=0.2  ic=0  Ts=0
  Scope : Scope  NumInputPorts=5
  Sum : Sum  Inputs=++++++
  Triggered Subsystem : Subsystem  TreatAsAtomicUnit=on
  Triggered Subsystem1 : Subsystem  TreatAsAtomicUnit=on
  safeErrors : Subsystem
  safeErrors1 : Subsystem
  safeErrors2 : Subsystem
  steadyState : Subsystem
  state : Outport  InitialOutput=0  VectorParamsAs1DForOutWhenUnconnected=off
  wires:
  u/1 -> steadyState/1(u)
  AND1/1 -> AND/1, AND2/1  "steady state"
  steadyState/1(ssFlag) -> AND1/1
  safeErrors2/1(safetyFlag) -> AND2/2
  Triggered Subsystem1/1(Out1) -> Memory/1
  NOT1/1 -> On Delay1/1
  On Delay/1 -> AND2/3
  extraSpace/1 -> On Delay/1, NOT1/1
  safeErrors1/1(safetyFlag) -> AND1/2
  AND2/1 -> Triggered Subsystem1/Trigger
  On Delay1/1 -> AND/2
  followerErrors/1 -> safeErrors/1(errors)
  errors/1 -> safeErrors1/1(errors)
  virtualErrors/1 -> safeErrors2/1(errors)
  Triggered Subsystem/1(Out1) -> Sum/6
  canStartLC/1 -> AND5/2
  lcDone/1 -> AND6/2
  AND7/1 -> Scope/5, Triggered Subsystem/Trigger
  Data Type Conversion/1 -> Sum/1
  AND/1 -> AND7/2
  AND6/1 -> AND7/1, Sum/5, Scope/4
  Constant/1 -> AND3/1, Data Type Conversion/1
  AND5/1 -> Sum/4, Scope/3, AND6/1
  AND3/1 -> Sum/2, Scope/1, AND4/1
  Sum/1 -> state/1
  safeErrors/1(safetyFlag) -> AND4/2
  AND4/1 -> Sum/3, Scope/2, AND5/1
  Memory/1 -> AND3/2

== system full_maneuver_single_veh/Fd_bkp/Platoon Gap Generation Management ==
  posInPlatoon : Inport
  strategy : Inport  Port=2
  platoonState : Inport  Port=3
  Enable : EnablePort
  Scope : Scope  NumInputPorts=2
  assignExtraSpace : MATLAB Function  TreatAsAtomicUnit=on
  assignvirtualLeader : MATLAB Function  TreatAsAtomicUnit=on
  assignVL : Outport  VectorParamsAs1DForOutWhenUnconnected=off
  extraSpace : Outport  Port=2  VectorParamsAs1DForOutWhenUnconnected=off
  wires:
  assignvirtualLeader/1(virtualLeaderFlag) -> assignVL/1, Scope/1
  platoonState/1 -> assignExtraSpace/3(platoonState), assignvirtualLeader/3(platoonState)
  posInPlatoon/1 -> assignExtraSpace/2(posInPlatoon), assignvirtualLeader/2(posInPlatoon)
  strategy/1 -> assignExtraSpace/1(strategy), assignvirtualLeader/1(strategy)
  assignExtraSpace/1(extraSpaceFlag) -> extraSpace/1, Scope/2

== system full_maneuver_single_veh/Fd_bkp/Platoon LC Management ==
  platoonStates : Inport
  strategy : Inport  Port=2
  Compare To Constant : simulink/Logic and Bit Operations/Compare To Constant  relop=>  const=1  OutDataTypeStr=boolean
  Compare To Constant1 : simulink/Logic and Bit Operations/Compare To Constant  relop=>  const=2  OutDataTypeStr=boolean
  OR : Logic  Operator=OR  IconShape=distinctive  AllPortsSameDT=off  OutDataTypeStr=boolean
  Selector : Selector  IndexOptions=Index vector (port)  Indices=[1 3]  OutputSizes=1
  Width : Width
  Out1 : Outport  VectorParamsAs1DForOutWhenUnconnected=off
  wires:
  Compare To Constant1/1 -> OR/1
  Selector/1 -> Compare To Constant1/1
  Width/1 -> Selector/2
  platoonStates/1 -> Selector/1, Width/1
  OR/1 -> Out1/1
  Compare To Constant/1 -> OR/2
  strategy/1 -> Compare To Constant/1

== system full_maneuver_single_veh/Fd_bkp/Regular Vehicle Following ==
  ego : Inport
  leader : Inport  Port=2
  leaderChange : Inport  Port=3
  extraSpaceFlag : Inport  Port=4
  Bus Selector : BusSelector  OutputSignals=Xdot,xddot
  Compute Errors : Subsystem
  Constant : Constant  Value=0
  Define Desired Distance : Subsystem
  Gain : Gain  Gain=-1
  Rate Limiter : RateLimiter  RisingSlewLimit=maxJerk  FallingSlewLimit=minJerk  SampleTimeMode=inherited
  Rate Limiter1 : RateLimiter  RisingSlewLimit=maxComfJerk  FallingSlewLimit=minComfJerk  SampleTimeMode=inherited
  Sum : Sum  Inputs=+-|
  Switch : Switch  Criteria=u2 > Threshold
  Switch1 : Switch  Criteria=u2 > Threshold
  Veh Following : Subsystem  TreatAsAtomicUnit=on
  Velocity Control : Subsystem  TreatAsAtomicUnit=on
  comf saturation : Saturate  UpperLimit=maxComfAccel  LowerLimit=minComfAccel
  errorScope : Scope
  freeFlowVel : Constant  Value=freeFlowVel
  safe saturation : Saturate  UpperLimit=maxAcceleration  LowerLimit=minAcceleration
  switch free flow : Subsystem
  veh foll state : Scope  NumInputPorts=2
  u : Outport  VectorParamsAs1DForOutWhenUnconnected=off
  errors : Outport  Port=2  VectorParamsAs1DForOutWhenUnconnected=off
  gap : Outport  Port=3  VectorParamsAs1DForOutWhenUnconnected=off
  leaderInRange : Outport  Port=4  VectorParamsAs1DForOutWhenUnconnected=off
  wires:
  Veh Following/1(u) -> Switch/1
  Constant/1 -> Compute Errors/5(velFilterReset)
  leaderChange/1 -> Veh Following/4(leaderChange)
  leader/1 -> Compute Errors/2(leader)
  switch free flow/1(inRange) -> Veh Following/5(inRange), veh foll state/1, Switch/2, leaderInRange/1
  Compute Errors/1(errors) -> Veh Following/1(errors), switch free flow/1(errors), errors/1, errorScope/1
  comf saturation/1 -> Rate Limiter1/1
  safe saturation/1 -> Rate Limiter/1
  Rate Limiter/1 -> Switch1/1  "sat(u)"
  Switch1/1 -> u/1
  Switch/1 -> veh foll state/2, safe saturation/1, comf saturation/1
  Rate Limiter1/1 -> Switch1/3  "sat(u)"
  Compute Errors/3("gap ") -> gap/1, switch free flow/3(gap)
  ego/1 -> Bus Selector/1, Compute Errors/1(ego)
  Bus Selector/1 -> Sum/2  "<Xdot>"
  Velocity Control/1(u) -> Switch/3
  freeFlowVel/1 -> Sum/1, switch free flow/6(vRef)
  Sum/1 -> Velocity Control/1(ev)
  Compute Errors/4(unsafeFlag) -> Switch1/2
  Bus Selector/2 -> Velocity Control/3(realInput), Veh Following/3(realInput), Gain/1  "<xddot>"
  Gain/1 -> Velocity Control/2(ea)
  Compute Errors/2(errorsDot) -> Veh Following/2(errorsDot), switch free flow/2(errorsDot)
  extraSpaceFlag/1 -> Define Desired Distance/1(extraSpaceFlag)
  Define Desired Distance/1(h) -> Compute Errors/3(h), switch free flow/4(h)
  Define Desired Distance/2(d0) -> Compute Errors/4(d0), switch free flow/5(d0)

== system full_maneuver_single_veh/Fd_bkp/Subsystem ==
  state : Inport
  u : Inport  Port=2
  Compare To Constant : simulink/Logic and Bit Operations/Compare To Constant  relop===  const=7  OutDataTypeStr=boolean
  Scope : Scope
  Switch1 : Switch  Criteria=u2 > Threshold
  comf saturation : Saturate  UpperLimit=maxComfAccel  LowerLimit=minComfAccel
  comf jerk : RateLimiter  RisingSlewLimit=maxComfJerk  FallingSlewLimit=minComfJerk  SampleTimeMode=inherited
  safe saturation : Saturate  UpperLimit=maxAcceleration  LowerLimit=minAcceleration
  safe jerk : RateLimiter  RisingSlewLimit=maxJerk  FallingSlewLimit=minJerk  SampleTimeMode=inherited
  sat(u) : Outport  VectorParamsAs1DForOutWhenUnconnected=off
  wires:
  safe saturation/1 -> safe jerk/1
  safe jerk/1 -> Switch1/1
  comf saturation/1 -> comf jerk/1
  state/1 -> Compare To Constant/1
  u/1 -> comf saturation/1, safe saturation/1
  comf jerk/1 -> Switch1/3
  Switch1/1 -> Scope/1, sat(u)/1
  Compare To Constant/1 -> Switch1/2

== system full_maneuver_single_veh/Fd_bkp/Triggered Subsystem ==
  Trigger : TriggerPort  VariantControl=Variant
  Constant : Constant
  lcFlag : Outport  InitialOutput=0  VectorParamsAs1DForOutWhenUnconnected=off
  wires:
  Constant/1 -> lcFlag/1

== system full_maneuver_single_veh/Fd_bkp/Virtual Follower Manager ==
  all : Inport
  posInPlatoon : Inport  Port=2
  lcStrategy : Inport  Port=3
  Enable : EnablePort
  Selector1 : Selector  InputPortWidth=5  IndexOptions=Index vector (port)  Indices=[1]  OutputSizes=1
  Width : Width
  determineVirtualFollower : MATLAB Function  TreatAsAtomicUnit=on
  virtualFollower : Outport
  wires:
  Width/1 -> determineVirtualFollower/1(nVehicles)
  lcStrategy/1 -> determineVirtualFollower/3(lcStrategy)
  determineVirtualFollower/1(virtualFollowerIdx) -> Selector1/2
  posInPlatoon/1 -> determineVirtualFollower/2(posInPlatoon)
  all/1 -> Selector1/1, Width/1
  Selector1/1 -> virtualFollower/1

== system full_maneuver_single_veh/Fd_bkp/Virtual Leader Manager ==
  all : Inport
  lcFlag : Inport  Port=2
  lcDone : Inport  Port=3
  posInPlatoon : Inport  Port=4
  lcStrategy : Inport  Port=5
  Enable : EnablePort
  Detect Change : simulink/Logic and Bit Operations/Detect Change  vinit=0  OutDataTypeStr=boolean
  Selector : Selector  InputPortWidth=5  IndexOptions=Index vector (port)  Indices=[1]  OutputSizes=1
  Width : Width
  determineVirtualLeader : MATLAB Function  TreatAsAtomicUnit=on
  virtualVehs : Scope
  virtualLeader : Outport  VectorParamsAs1DForOutWhenUnconnected=off
  leaderChange : Outport  Port=2  VectorParamsAs1DForOutWhenUnconnected=off
  wires:
  all/1 -> Selector/1, Width/1
  Selector/1 -> virtualLeader/1
  Detect Change/1 -> leaderChange/1
  determineVirtualLeader/1(virtualLeaderIdx) -> Selector/2, Detect Change/1, virtualVehs/1
  Width/1 -> determineVirtualLeader/1(nVehicles)
  lcFlag/1 -> determineVirtualLeader/2(lcFlag)
  lcDone/1 -> determineVirtualLeader/3(lcDone)
  posInPlatoon/1 -> determineVirtualLeader/4(posInPlatoon)
  lcStrategy/1 -> determineVirtualLeader/5(lcStrategy)

== system full_maneuver_single_veh/Fd_bkp/Virtual Vehicle Following ==
  ego : Inport
  virtualLeader : Inport  Port=2
  leaderChange : Inport  Port=3
  extraSpaceFlag : Inport  Port=4
  Enable : EnablePort
  AND : Logic  IconShape=distinctive  AllPortsSameDT=off  OutDataTypeStr=boolean
  Bus Selector : BusSelector  OutputSignals=Xdot,xddot
  Chart : Stateflow chart  TreatAsAtomicUnit=on
  Compute Errors : Subsystem
  Define Desired Distance : Subsystem
  Gain : Gain  Gain=-1
  Gain1 : Gain  Gain=-1
  NOT : Logic  Operator=NOT  IconShape=distinctive  AllPortsSameDT=off  OutDataTypeStr=boolean
  Scope : Scope  NumInputPorts=2
  Scope1 : Scope  NumInputPorts=2
  Sum : Sum  Inputs=|+-
  Sum6 : Sum  Inputs=|+-
  Terminator : Terminator
  Velocity Control1 : Subsystem  TreatAsAtomicUnit=on
  Velocity Control2 : Subsystem  TreatAsAtomicUnit=on
  Virtual Leader Following : Subsystem  TreatAsAtomicUnit=on
  freeFlowVel : Constant  Value=freeFlowVel
  switch free flow : Subsystem
  switch min vel : Subsystem
  vMin : Constant  Value=vMin
  u : Outport  InitialOutput=0  VectorParamsAs1DForOutWhenUnconnected=off
  virtualErrors : Outport  Port=2  OutputWhenDisabled=reset  InitialOutput=[0, 0]  VectorParamsAs1DForOutWhenUnconnected=off
  virtualGap : Outport  Port=3  OutputWhenDisabled=reset  InitialOutput=[0]  VectorParamsAs1DForOutWhenUnconnected=off
  vLeaderFarAhead : Outport  Port=4  VectorParamsAs1DForOutWhenUnconnected=off
  wires:
  NOT/1 -> Chart/3(leaderInRangeBehind), AND/2
  switch min vel/1(inRange) -> NOT/1
  extraSpaceFlag/1 -> Define Desired Distance/1(extraSpaceFlag)
  Velocity Control1/1(u) -> Chart/5(uMinVelControl)  "uMinVelControl"
  Chart/1(state) -> Scope/1
  Compute Errors/3("gap ") -> virtualGap/1, switch min vel/3(gap), switch free flow/3(gap)
  Bus Selector/1 -> Scope1/1, Sum/2, Sum6/2  "<Xdot>"
  Virtual Leader Following/1(u) -> Chart/1(uVehFoll)  "uVehFoll"
  ego/1 -> Compute Errors/1(ego), Bus Selector/1
  vMin/1 -> switch min vel/6(vRef), Scope1/2, Sum/1
  Compute Errors/1(errors) -> switch min vel/1(errors), switch free flow/1(errors), Virtual Leader Following/1(errors), virtualErrors/1
  virtualLeader/1 -> Compute Errors/2(leader)
  Sum6/1 -> Velocity Control2/1(ev)
  Chart/2(u) -> Scope/2, u/1
  freeFlowVel/1 -> Sum6/1, switch free flow/6(vRef)
  Sum/1 -> Velocity Control1/1(ev)
  Velocity Control2/1(u) -> Chart/4(uFreeFlowVelControl)  "uFreeFlowControl"
  switch free flow/1(inRange) -> vLeaderFarAhead/1, Chart/2(leaderInRange), AND/1
  leaderChange/1 -> Compute Errors/5(velFilterReset), Virtual Leader Following/4(leaderChange)
  Compute Errors/4(unsafeFlag) -> Terminator/1
  Bus Selector/2 -> Velocity Control1/3(realInput), Virtual Leader Following/3(realInput), Gain/1, Velocity Control2/3(realInput), Gain1/1  "<xddot>"
  Compute Errors/2(errorsDot) -> switch min vel/2(errorsDot), switch free flow/2(errorsDot), Virtual Leader Following/2(errorsDot)
  Gain/1 -> Velocity Control2/2(ea)
  Gain1/1 -> Velocity Control1/2(ea)
  Define Desired Distance/1(h) -> switch min vel/4(h), switch free flow/4(h), Compute Errors/3(h)
  Define Desired Distance/2(d0) -> switch min vel/5(d0), switch free flow/5(d0), Compute Errors/4(d0)
  AND/1 -> Virtual Leader Following/5(inRange)

== system full_maneuver_single_veh/Fd_bkp/lateral steady state ==
  u : Inport
  AND : Logic  IconShape=distinctive  AllPortsSameDT=off  OutDataTypeStr=boolean
  Abs2 : Abs
  Compare To Constant2 : simulink/Logic and Bit Operations/Compare To Constant  relop=<=  const=0.2  OutDataTypeStr=boolean
  Demux : Demux  Outputs=2
  Mux : Mux  Inputs=2
  Transport Delay2 : TransportDelay
  ssFlag : Outport  VectorParamsAs1DForOutWhenUnconnected=off
  wires:
  u/1 -> Transport Delay2/1, Mux/2
  Abs2/1 -> Compare To Constant2/1
  Demux/1 -> AND/1
  Transport Delay2/1 -> Mux/1
  AND/1 -> ssFlag/1
  Compare To Constant2/1 -> Demux/1
  Mux/1 -> Abs2/1
  Demux/2 -> AND/2

== system full_maneuver_single_veh/Fd_bkp/states routing ==
  delta : Inport
  Info : Inport  Port=2
  u : Inport  Port=3
  Bus Creator : BusCreator  Inputs=7  OutDataTypeStr=Bus: vehStatesBus  NonVirtualBus=on
      settings: InheritFromInputs=off
  Bus Selector : BusSelector  OutputSignals=BdyFrm.Cg.Vel.ydot,BdyFrm.Cg.AngVel.r,InertFrm.RearAxl.Disp.X,InertFrm.Cg.Disp.Y,InertFrm.RearAxl.Vel.Xdot,BdyFrm.Cg.Acc.xddot,InertFrm.Cg.Ang.psi
  Mux : Mux
  latStates : Outport
  observedStates : Outport  Port=2
  wires:
  Bus Creator/1 -> observedStates/1
  Bus Selector/2 -> Mux/4  "<r>"
  Bus Selector/1 -> Mux/2  "<ydot>"
  Mux/1 -> latStates/1
  delta/1 -> Bus Creator/7
  u/1 -> Bus Creator/6
  Bus Selector/7 -> Mux/3, Bus Creator/5  "<psi>"
  Bus Selector/6 -> Bus Creator/4  "<xddot>"
  Bus Selector/5 -> Bus Creator/3  "<Xdot>"
  Bus Selector/4 -> Mux/1, Bus Creator/2  "<Y>"
  Bus Selector/3 -> Bus Creator/1  "<X>"
  Info/1 -> Bus Selector/1
